simulink model "pmsm_control"  (R2018b)
settings: Solver=FixedStepDiscrete  StartTime=0.0  StopTime=0.5  FixedStep=dt_plant_sim  RelTol=1e-6  EnableMultiTasking=on
InitFcn:
  | pmsm_control_init
values from neighbouring files (symbols this model uses):
  D_safe = Simulink.Parameter(single(D0))    [pmsm_control_init.m]
  dt = 50e-9    (= 5e-08)    [pmsm_init.m]
  I_limit = Simulink.Parameter(single(Imax))    [pmsm_control_init.m]
  Id_Ki = Simulink.Parameter(single((Id_Kp.Value / TI) * Ts_current))    [pmsm_control_init.m]
  Id_Kp = Simulink.Parameter(single(wc * Ld))    [pmsm_control_init.m]
  ImaxFX = 600    [pmsm_init.m]
  Iq_Ki = Simulink.Parameter(single((Iq_Kp.Value / TI) * Ts_current))    [pmsm_control_init.m]
  Iq_Kp = Simulink.Parameter(single(wc * Lq))    [pmsm_control_init.m]
  J = Tst*Tau/W    (= 0.15)    [pmsm_init.m]
  L = Ld    [pmsm_control_init.m]    (also in pmsm_init.m = [Ld Lq])
  Ld = 0.37e-3    (= 0.00037)    [pmsm_init.m]
  Lq = 1.2e-3    (= 0.0012)    [pmsm_init.m]
  modulation_limit = Simulink.Parameter(single(0.577350269189626))    [pmsm_control_init.m]
  open_loop_iq_ref = Simulink.Parameter(single(5))    [pmsm_control_init.m]
  open_loop_mode = Simulink.Parameter(boolean(0))    [pmsm_control_init.m]
  pp = 3    [pmsm_init.m]
  Psi_PM = 66e-3    (= 0.066)    [pmsm_init.m]
  PsimaxFX = 2*abs(Psi_PM + Ld*Imax + j*Lq*Imax)    [pmsm_init.m]
  PWM_it_period = Simulink.Parameter(2)    [pmsm_control_init.m]
  R = 18e-3    (= 0.018)    [pmsm_init.m]
  Speed_Iq_limit = Simulink.Parameter(single(40))    [pmsm_control_init.m]
  Speed_Ki = Simulink.Parameter(single(Speed_Kp.Value / 0.03))    [pmsm_control_init.m]
  Speed_Kp = Simulink.Parameter(single(0.4))    [pmsm_control_init.m]
  TaumaxFX = (3/2)*pp*real(j*(Psi_PM + Ld*Imax + j*Lq*Imax)*Imax*(-1+j))    [pmsm_init.m]
  Ts = 1 / fsw    (= 0.0001)    [pmsm_control_init.m]
  Ts_current = Ts    (= 0.0001)    [pmsm_control_init.m]
  Ub = Udc / 2    [pmsm_control_init.m]
  Udc = 300    [pmsm_init.m]
  Udc_min = Simulink.Parameter(single(20))    [pmsm_control_init.m]
  UmaxFX = 600    [pmsm_init.m]
  WmaxFX = 1500*pp    (= 4500)    [pmsm_init.m]
undefined symbols (not defined in the file or in its folder): DiscIntNeverNeededParam, j
libraries: simulink x7
settings Model: ModifiedByFormat=The MathWorks Inc.  Creator=The MathWorks, Inc.  LastModifiedBy=The MathWorks Inc.
settings DataIOCC: LimitDataPoints=on  SaveFormat=Array  SaveOutput=off  SaveTime=off
settings OptimizationCC: ExpressionDepthLimit=2147483647  LifeSpan=1
settings DebuggingCC: MergeDetectMultiDrivingBlocksExec=none  SolverPrmCheckMsg=warning  FcnCallInpInsideContextMsg=warning  StateNameClashWarn=warning  SFUnexpectedBacktrackingDiag=warning  SFNoUnconditionalDefaultTransitionDiag=warning  SFExecutionAtInitializationDiag=none
settings HardwareCC: ProdBitPerPointer=32  ProdBitPerSizeT=32  ProdBitPerPtrDiffT=32  ProdLargestAtomicFloat=None  ProdIntDivRoundTo=Undefined  ProdEndianess=Unspecified  ProdWordSize=32  ProdHWDeviceType=32-bit Generic
settings ModelReferenceCC: PropagateSignalLabelsOutOfModel=off
settings SFSimCC: SimUseLocalCustomCode=off
settings RTWCC: RTWUseLocalCustomCode=off
settings CodeAppCC: StateflowObjectComments=on
settings GRTTargetCC: TargetLangStandard=C89/C90 (ANSI)  CombineOutputUpdateFcns=off  GRTInterface=on
settings ConfigComp: CovMetricSettings=dw  CovSaveCumulativeToWorkspaceVar=on  CovSaveSingleToWorkspaceVar=on  CovExternalEMLEnable=off  CovSFcnEnable=off

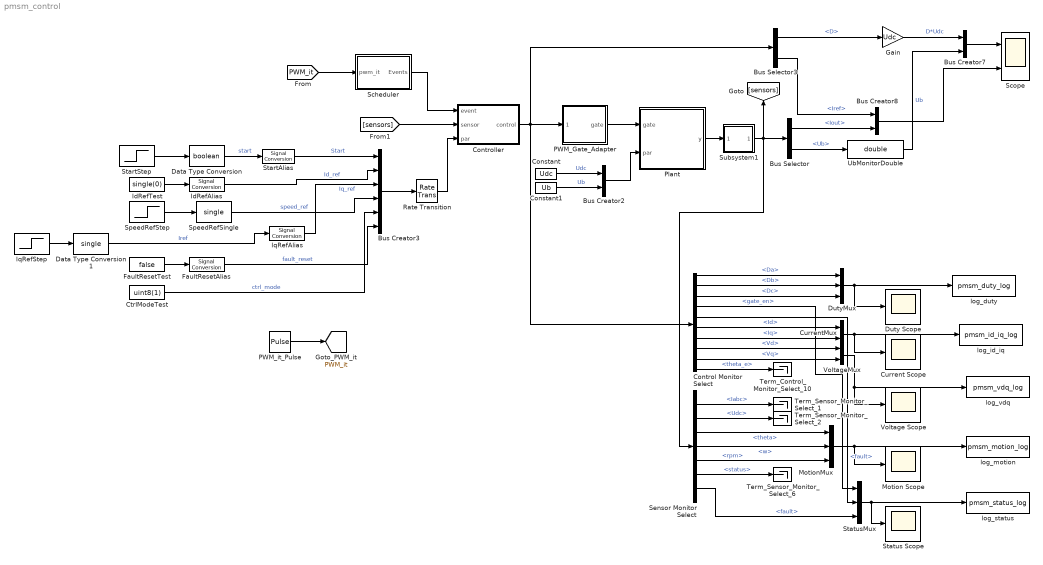
== system pmsm_control ==
  Bus Creator2 : BusCreator  Inputs=2
  Bus Creator3 : BusCreator  Inputs=6
  Bus Creator7 : BusCreator  Inputs=2
  Bus Creator8 : BusCreator  Inputs=2
  Bus Selector : BusSelector  OutputSignals=Iout,Ub
  Bus Selector3 : BusSelector  OutputSignals=D,Iref
  Constant : Constant  Value=Udc  SampleTime=-1
  Constant1 : Constant  Value=Ub  SampleTime=-1
  Control Monitor Select : BusSelector  OutputSignals=Da,Db,Dc,gate_en,fault,Id,Iq,Vd,Vq,theta_e
  Controller : Subsystem
  CtrlModeTest : Constant  Value=uint8(1)  OutDataTypeStr=uint8
  Current Scope : Scope
  CurrentMux : Mux  Inputs=2
  Data Type Conversion : DataTypeConversion  OutDataTypeStr=boolean
  Data Type Conversion1 : DataTypeConversion  OutDataTypeStr=single
  Duty Scope : Scope
  DutyMux : Mux  Inputs=3
  FaultResetAlias : SignalConversion  OverrideOpt=off
  FaultResetTest : Constant  Value=false  OutDataTypeStr=boolean
  Gain : Gain  Gain=Udc  ParamDataTypeStr=double  OutDataTypeStr=double
  IdRefAlias : SignalConversion  OverrideOpt=off
  IdRefTest : Constant  Value=single(0)  OutDataTypeStr=single
  IqRefAlias : SignalConversion  OverrideOpt=off
  IqRefStep : Step  Time=0  After=20  SampleTime=0
  Motion Scope : Scope
  MotionMux : Mux  Inputs=3
  PWM_Gate_Adapter : Subsystem
  PWM_it_Pulse : DiscretePulseGenerator  Period=PWM_it_period  SampleTime=Ts_current/2
  Plant : Subsystem
  Rate Transition : RateTransition  Integrity=off  Deterministic=off
  Scheduler : Subsystem
  Scope : Scope  NumInputPorts=2
  Sensor Monitor Select : BusSelector  OutputSignals=Iabc,Udc,theta,w,rpm,status,fault
  SpeedRefSingle : DataTypeConversion  OutDataTypeStr=single
  SpeedRefStep : Step  Time=0  Before=100  After=100  SampleTime=0
  StartAlias : SignalConversion  OverrideOpt=off
  StartStep : Step  Time=0  SampleTime=0
  Status Scope : Scope
  StatusMux : Mux  Inputs=3
  Subsystem1 : Subsystem
  Term_Control_Monitor_Select_10 : Terminator
  Term_Sensor_Monitor_Select_1 : Terminator
  Term_Sensor_Monitor_Select_2 : Terminator
  Term_Sensor_Monitor_Select_6 : Terminator
  UbMonitorDouble : DataTypeConversion  OutDataTypeStr=double
  Voltage Scope : Scope
  VoltageMux : Mux  Inputs=2
  log_duty : ToWorkspace  VariableName=pmsm_duty_log  SaveFormat=Structure With Time  SampleTime=-1
  log_id_iq : ToWorkspace  VariableName=pmsm_id_iq_log  SaveFormat=Structure With Time  SampleTime=-1
  log_motion : ToWorkspace  VariableName=pmsm_motion_log  SaveFormat=Structure With Time  SampleTime=-1
  log_status : ToWorkspace  VariableName=pmsm_status_log  SaveFormat=Structure With Time  SampleTime=-1
  log_vdq : ToWorkspace  VariableName=pmsm_vdq_log  SaveFormat=Structure With Time  SampleTime=-1
  tag scope: PWM_it=global
  wires:
  Constant/1 -> Bus Creator2/1  "Udc"
  Constant1/1 -> Bus Creator2/2  "Ub"
  Bus Selector3/1 -> Gain/1  "<D>"
  Gain/1 -> Bus Creator7/1  "D*Udc"
  Bus Selector3/2 -> Bus Creator8/1  "<Iref>"
  Bus Selector/1 -> Bus Creator8/2  "<Iout>"
  Bus Creator7/1 -> Scope/1
  Bus Creator8/1 -> Scope/2
  Scheduler/1(Events) -> Controller/1(event)
  Data Type Conversion/1 -> StartAlias/1  "start"
  Data Type Conversion1/1 -> IqRefAlias/1  "Iref"
  Bus Creator3/1 -> Rate Transition/1
  [sensors] -> Controller/2(sensor)
  Subsystem1/1(Out1) -> Sensor Monitor Select/1, Bus Selector/1, [sensors]
  Rate Transition/1 -> Controller/3(par)
  [PWM_it] -> Scheduler/1(pwm_it)
  IdRefTest/1 -> IdRefAlias/1
  FaultResetTest/1 -> FaultResetAlias/1
  DutyMux/1 -> log_duty/1, Duty Scope/1
  CurrentMux/1 -> Current Scope/1, log_id_iq/1
  VoltageMux/1 -> Voltage Scope/1, log_vdq/1
  MotionMux/1 -> Motion Scope/1, log_motion/1
  StatusMux/1 -> Status Scope/1, log_status/1
  StartStep/1 -> Data Type Conversion/1
  IqRefStep/1 -> Data Type Conversion1/1
  Control Monitor Select/1 -> DutyMux/1  "<Da>"
  Control Monitor Select/2 -> DutyMux/2  "<Db>"
  Control Monitor Select/3 -> DutyMux/3  "<Dc>"
  Control Monitor Select/6 -> CurrentMux/1  "<Id>"
  Control Monitor Select/7 -> CurrentMux/2  "<Iq>"
  Control Monitor Select/8 -> VoltageMux/1  "<Vd>"
  Control Monitor Select/9 -> VoltageMux/2  "<Vq>"
  Sensor Monitor Select/3 -> MotionMux/1  "<theta>"
  Sensor Monitor Select/4 -> MotionMux/2  "<w>"
  Sensor Monitor Select/5 -> MotionMux/3  "<rpm>"
  Control Monitor Select/4 -> StatusMux/1  "<gate_en>"
  Control Monitor Select/5 -> StatusMux/2  "<fault>"
  Sensor Monitor Select/7 -> StatusMux/3  "<fault>"
  Bus Selector/2 -> UbMonitorDouble/1  "<Ub>"
  UbMonitorDouble/1 -> Bus Creator7/2  "Ub"
  Controller/1(control) -> PWM_Gate_Adapter/1(control), Bus Selector3/1, Control Monitor Select/1
  Control Monitor Select/10 -> Term_Control_Monitor_Select_10/1  "<theta_e>"
  Sensor Monitor Select/1 -> Term_Sensor_Monitor_Select_1/1  "<Iabc>"
  Sensor Monitor Select/2 -> Term_Sensor_Monitor_Select_2/1  "<Udc>"
  Sensor Monitor Select/6 -> Term_Sensor_Monitor_Select_6/1  "<status>"
  PWM_Gate_Adapter/1(gate) -> Plant/1(gate)
  Bus Creator2/1 -> Plant/2(par)
  Plant/1(y) -> Subsystem1/1(In1)
  StartAlias/1 -> Bus Creator3/1  "Start"
  IdRefAlias/1 -> Bus Creator3/2  "Id_ref"
  IqRefAlias/1 -> Bus Creator3/3  "Iq_ref"
  FaultResetAlias/1 -> Bus Creator3/6  "fault_reset"
  PWM_it_Pulse/1 -> [PWM_it]
  SpeedRefStep/1 -> SpeedRefSingle/1
  SpeedRefSingle/1 -> Bus Creator3/4  "speed_ref"
  CtrlModeTest/1 -> Bus Creator3/5  "ctrl_mode"

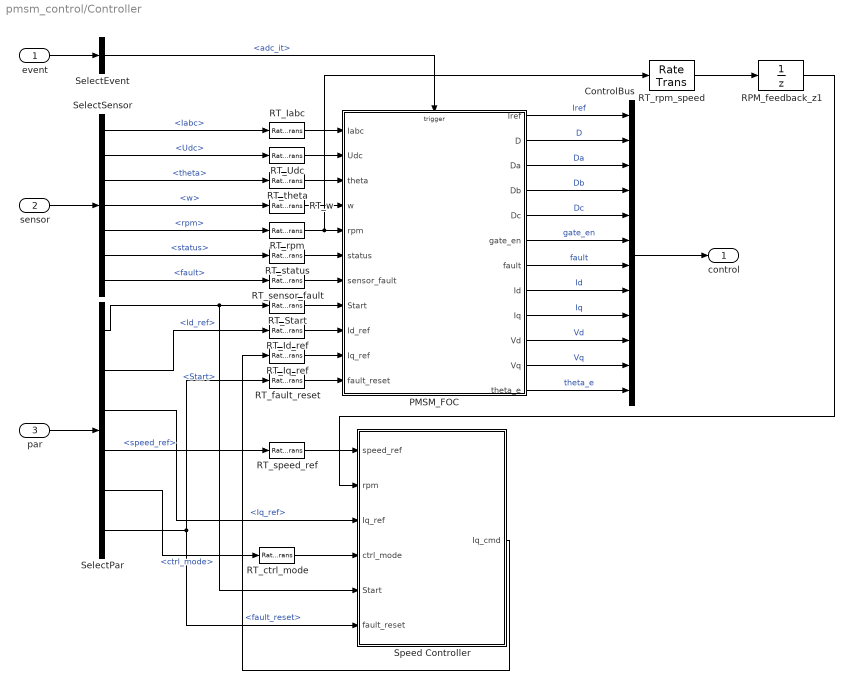
== system pmsm_control/Controller ==
  event : Inport
  sensor : Inport  Port=2
  par : Inport  Port=3
  ControlBus : BusCreator  Inputs=12
  PMSM_FOC : Subsystem  TreatAsAtomicUnit=on
  RPM_feedback_z1 : UnitDelay  InitialCondition=single(0)  SampleTime=-1
  RT_Iabc : RateTransition  Integrity=off  Deterministic=off  OutPortSampleTimeOpt=Inherit
  RT_Id_ref : RateTransition  Integrity=off  Deterministic=off  OutPortSampleTimeOpt=Inherit
  RT_Iq_ref : RateTransition  Integrity=off  Deterministic=off  OutPortSampleTimeOpt=Inherit
  RT_Start : RateTransition  Integrity=off  Deterministic=off  OutPortSampleTimeOpt=Inherit
  RT_Udc : RateTransition  Integrity=off  Deterministic=off  OutPortSampleTimeOpt=Inherit
  RT_ctrl_mode : RateTransition  Integrity=off  Deterministic=off  OutPortSampleTimeOpt=Inherit
  RT_fault_reset : RateTransition  Integrity=off  Deterministic=off  OutPortSampleTimeOpt=Inherit
  RT_rpm : RateTransition  Integrity=off  Deterministic=off  OutPortSampleTimeOpt=Inherit
  RT_rpm_speed : RateTransition  Deterministic=off  OutPortSampleTimeOpt=Inherit
  RT_sensor_fault : RateTransition  Integrity=off  Deterministic=off  OutPortSampleTimeOpt=Inherit
  RT_speed_ref : RateTransition  Integrity=off  Deterministic=off  OutPortSampleTimeOpt=Inherit
  RT_status : RateTransition  Integrity=off  Deterministic=off  OutPortSampleTimeOpt=Inherit
  RT_theta : RateTransition  Integrity=off  Deterministic=off  OutPortSampleTimeOpt=Inherit
  RT_w : RateTransition  Integrity=off  Deterministic=off  OutPortSampleTimeOpt=Inherit
  SelectEvent : BusSelector  OutputSignals=interrupts.adc_it
  SelectPar : BusSelector  OutputSignals=Start,Id_ref,Iq_ref,speed_ref,ctrl_mode,fault_reset
  SelectSensor : BusSelector  OutputSignals=Iabc,Udc,theta,w,rpm,status,fault
  Speed Controller : Subsystem
  control : Outport
  wires:
  RPM_feedback_z1/1 -> Speed Controller/2(rpm)
  RT_rpm_speed/1 -> RPM_feedback_z1/1
  PMSM_FOC/12(theta_e) -> ControlBus/12  "theta_e"
  PMSM_FOC/11(Vq) -> ControlBus/11  "Vq"
  PMSM_FOC/10(Vd) -> ControlBus/10  "Vd"
  PMSM_FOC/9(Iq) -> ControlBus/9  "Iq"
  PMSM_FOC/8(Id) -> ControlBus/8  "Id"
  PMSM_FOC/7(fault) -> ControlBus/7  "fault"
  PMSM_FOC/6(gate_en) -> ControlBus/6  "gate_en"
  PMSM_FOC/5(Dc) -> ControlBus/5  "Dc"
  PMSM_FOC/4(Db) -> ControlBus/4  "Db"
  PMSM_FOC/3(Da) -> ControlBus/3  "Da"
  PMSM_FOC/2(D) -> ControlBus/2  "D"
  PMSM_FOC/1(Iref) -> ControlBus/1  "Iref"
  RT_fault_reset/1 -> PMSM_FOC/11(fault_reset)
  RT_Iq_ref/1 -> PMSM_FOC/10(Iq_ref)
  RT_Id_ref/1 -> PMSM_FOC/9(Id_ref)
  RT_Start/1 -> PMSM_FOC/8(Start)
  RT_sensor_fault/1 -> PMSM_FOC/7(sensor_fault)
  RT_status/1 -> PMSM_FOC/6(status)
  RT_rpm/1 -> RT_rpm_speed/1, PMSM_FOC/5(rpm)
  RT_w/1 -> PMSM_FOC/4(w)
  RT_theta/1 -> PMSM_FOC/3(theta)
  RT_Udc/1 -> PMSM_FOC/2(Udc)
  RT_Iabc/1 -> PMSM_FOC/1(Iabc)
  ControlBus/1 -> control/1
  SelectSensor/7 -> RT_sensor_fault/1  "<fault>"
  SelectSensor/6 -> RT_status/1  "<status>"
  SelectSensor/5 -> RT_rpm/1  "<rpm>"
  SelectSensor/4 -> RT_w/1  "<w>"
  SelectSensor/3 -> RT_theta/1  "<theta>"
  SelectSensor/2 -> RT_Udc/1  "<Udc>"
  SelectSensor/1 -> RT_Iabc/1  "<Iabc>"
  SelectEvent/1 -> PMSM_FOC/Trigger  "<adc_it>"
  par/1 -> SelectPar/1
  sensor/1 -> SelectSensor/1
  event/1 -> SelectEvent/1
  SelectPar/1 -> Speed Controller/5(Start), RT_Start/1  "<Start>"
  SelectPar/2 -> RT_Id_ref/1  "<Id_ref>"
  SelectPar/3 -> Speed Controller/3(Iq_ref)  "<Iq_ref>"
  SelectPar/4 -> RT_speed_ref/1  "<speed_ref>"
  SelectPar/5 -> RT_ctrl_mode/1  "<ctrl_mode>"
  SelectPar/6 -> Speed Controller/6(fault_reset), RT_fault_reset/1  "<fault_reset>"
  RT_speed_ref/1 -> Speed Controller/1(speed_ref)
  RT_ctrl_mode/1 -> Speed Controller/4(ctrl_mode)
  Speed Controller/1(Iq_cmd) -> RT_Iq_ref/1

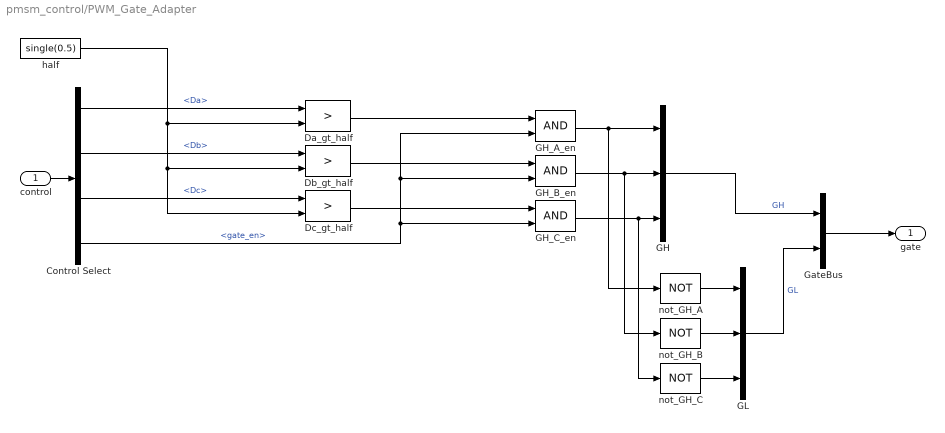
== system pmsm_control/PWM_Gate_Adapter ==
  control : Inport
  Control Select : BusSelector  OutputSignals=Da,Db,Dc,gate_en
  Da_gt_half : RelationalOperator  Operator=>  OutDataTypeStr=boolean  RndMeth=Simplest
  Db_gt_half : RelationalOperator  Operator=>  OutDataTypeStr=boolean  RndMeth=Simplest
  Dc_gt_half : RelationalOperator  Operator=>  OutDataTypeStr=boolean  RndMeth=Simplest
  GH : Mux  Inputs=3
  GH_A_en : Logic  AllPortsSameDT=off  OutDataTypeStr=boolean
  GH_B_en : Logic  AllPortsSameDT=off  OutDataTypeStr=boolean
  GH_C_en : Logic  AllPortsSameDT=off  OutDataTypeStr=boolean
  GL : Mux  Inputs=3
  GateBus : BusCreator  Inputs=2
  half : Constant  Value=single(0.5)  OutDataTypeStr=single
  not_GH_A : Logic  Operator=NOT  AllPortsSameDT=off  OutDataTypeStr=boolean
  not_GH_B : Logic  Operator=NOT  AllPortsSameDT=off  OutDataTypeStr=boolean
  not_GH_C : Logic  Operator=NOT  AllPortsSameDT=off  OutDataTypeStr=boolean
  gate : Outport
  wires:
  Control Select/1 -> Da_gt_half/1  "<Da>"
  half/1 -> Da_gt_half/2, Dc_gt_half/2, Db_gt_half/2
  Da_gt_half/1 -> GH_A_en/1
  Control Select/4 -> GH_A_en/2, GH_B_en/2, GH_C_en/2  "<gate_en>"
  GH_A_en/1 -> GH/1, not_GH_A/1
  Control Select/2 -> Db_gt_half/1  "<Db>"
  Db_gt_half/1 -> GH_B_en/1
  GH_B_en/1 -> GH/2, not_GH_B/1
  Control Select/3 -> Dc_gt_half/1  "<Dc>"
  Dc_gt_half/1 -> GH_C_en/1
  GH_C_en/1 -> not_GH_C/1, GH/3
  control/1 -> Control Select/1
  not_GH_A/1 -> GL/1
  not_GH_B/1 -> GL/2
  not_GH_C/1 -> GL/3
  GH/1 -> GateBus/1  "GH"
  GL/1 -> GateBus/2  "GL"
  GateBus/1 -> gate/1

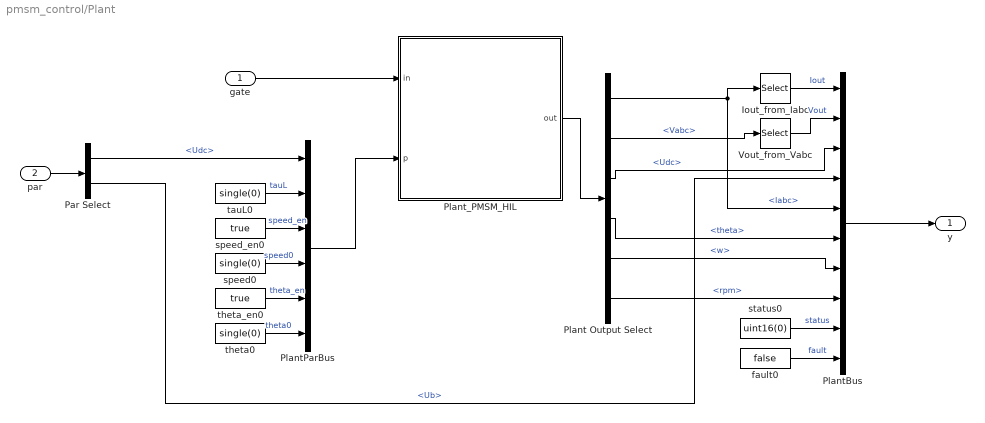
== system pmsm_control/Plant ==
  gate : Inport
  par : Inport  Port=2
  Iout_from_Iabc : Selector  InputPortWidth=3  IndexOptions=Index vector (dialog)  Indices=1  OutputSizes=1
  Par Select : BusSelector  OutputSignals=Udc,Ub
  Plant Output Select : BusSelector  OutputSignals=Iabc,Vabc,Udc,theta,w,rpm
  PlantBus : BusCreator  Inputs=10
  PlantParBus : BusCreator  Inputs=6
  Plant_PMSM_HIL : Subsystem
  Vout_from_Vabc : Selector  InputPortWidth=3  IndexOptions=Index vector (dialog)  Indices=1  OutputSizes=1
  fault0 : Constant  Value=false  OutDataTypeStr=boolean
  speed0 : Constant  Value=single(0)  OutDataTypeStr=single
  speed_en0 : Constant  Value=true  OutDataTypeStr=boolean
  status0 : Constant  Value=uint16(0)  OutDataTypeStr=uint16
  tauL0 : Constant  Value=single(0)  OutDataTypeStr=single
  theta0 : Constant  Value=single(0)  OutDataTypeStr=single
  theta_en0 : Constant  Value=true  OutDataTypeStr=boolean
  y : Outport
  wires:
  Par Select/1 -> PlantParBus/1  "<Udc>"
  tauL0/1 -> PlantParBus/2  "tauL"
  speed_en0/1 -> PlantParBus/3  "speed_en"
  speed0/1 -> PlantParBus/4  "speed0"
  theta_en0/1 -> PlantParBus/5  "theta_en"
  theta0/1 -> PlantParBus/6  "theta0"
  Plant Output Select/1 -> Iout_from_Iabc/1, PlantBus/5  "<Iabc>"
  Plant Output Select/2 -> Vout_from_Vabc/1  "<Vabc>"
  Iout_from_Iabc/1 -> PlantBus/1  "Iout"
  Vout_from_Vabc/1 -> PlantBus/2  "Vout"
  Plant Output Select/3 -> PlantBus/3  "<Udc>"
  Par Select/2 -> PlantBus/4  "<Ub>"
  Plant Output Select/4 -> PlantBus/6  "<theta>"
  Plant Output Select/5 -> PlantBus/7  "<w>"
  Plant Output Select/6 -> PlantBus/8  "<rpm>"
  status0/1 -> PlantBus/9  "status"
  fault0/1 -> PlantBus/10  "fault"
  gate/1 -> Plant_PMSM_HIL/1(in)
  par/1 -> Par Select/1
  PlantParBus/1 -> Plant_PMSM_HIL/2(p)
  Plant_PMSM_HIL/1(out) -> Plant Output Select/1
  PlantBus/1 -> y/1

== system pmsm_control/Scheduler ==
  pwm_it : Inport
  AsynchronousScheduler : Stateflow chart  TreatAsAtomicUnit=on
      settings: RTWMemSecFuncInitTerm=Default  RTWMemSecFuncExecute=Default
  Bus Creator : BusCreator  Inputs=1
  Bus Creator4 : BusCreator  Inputs=2
  Bus Creator5 : BusCreator  Inputs=3
  Function-Call Generator : simulink/Ports & Subsystems/Function-Call Generator  sample_time=1e-3  numberOfIterations=1
  Function-Call Generator1 : simulink/Ports & Subsystems/Function-Call Generator  sample_time=100e-3  numberOfIterations=1
  Function-Call Generator2 : simulink/Ports & Subsystems/Function-Call Generator  sample_time=1  numberOfIterations=1
  Events : Outport
  wires:
  Bus Creator5/1 -> Bus Creator4/2  "timers"
  Function-Call Generator2/1 -> Bus Creator5/3  "T_1s"
  Bus Creator/1 -> Bus Creator4/1  "interrupts"
  pwm_it/1 -> AsynchronousScheduler/Trigger  "pwm_it"
  AsynchronousScheduler/1(adc_it()) -> Bus Creator/1
  Bus Creator4/1 -> Events/1
  Function-Call Generator1/1 -> Bus Creator5/2  "T_100ms"
  Function-Call Generator/1 -> Bus Creator5/1  "T_1ms"

== system pmsm_control/Subsystem1 ==
  In1 : Inport
  Iabc_conv : DataTypeConversion  OutDataTypeStr=single
  Iout_conv : DataTypeConversion  OutDataTypeStr=single
  SelectPlant : BusSelector  OutputSignals=Iout,Vout,Udc,Ub,Iabc,theta,w,rpm,status,fault
  SensorBus : BusCreator  Inputs=10
  Ub_conv : DataTypeConversion  OutDataTypeStr=single
  Udc_conv : DataTypeConversion  OutDataTypeStr=single
  Vout_conv : DataTypeConversion  OutDataTypeStr=single
  fault_conv : DataTypeConversion  OutDataTypeStr=boolean
  rpm_conv : DataTypeConversion  OutDataTypeStr=single
  status_conv : DataTypeConversion  OutDataTypeStr=uint16
  theta_conv : DataTypeConversion  OutDataTypeStr=single
  w_conv : DataTypeConversion  OutDataTypeStr=single
  Out1 : Outport
  wires:
  In1/1 -> SelectPlant/1
  SelectPlant/1 -> Iout_conv/1  "<Iout>"
  Iout_conv/1 -> SensorBus/1  "Iout"
  SelectPlant/2 -> Vout_conv/1  "<Vout>"
  Vout_conv/1 -> SensorBus/2  "Vout"
  SelectPlant/3 -> Udc_conv/1  "<Udc>"
  Udc_conv/1 -> SensorBus/3  "Udc"
  SelectPlant/4 -> Ub_conv/1  "<Ub>"
  Ub_conv/1 -> SensorBus/4  "Ub"
  SelectPlant/5 -> Iabc_conv/1  "<Iabc>"
  Iabc_conv/1 -> SensorBus/5  "Iabc"
  SelectPlant/6 -> theta_conv/1  "<theta>"
  theta_conv/1 -> SensorBus/6  "theta"
  SelectPlant/7 -> w_conv/1  "<w>"
  w_conv/1 -> SensorBus/7  "w"
  SelectPlant/8 -> rpm_conv/1  "<rpm>"
  rpm_conv/1 -> SensorBus/8  "rpm"
  SelectPlant/9 -> status_conv/1  "<status>"
  status_conv/1 -> SensorBus/9  "status"
  SelectPlant/10 -> fault_conv/1  "<fault>"
  fault_conv/1 -> SensorBus/10  "fault"
  SensorBus/1 -> Out1/1

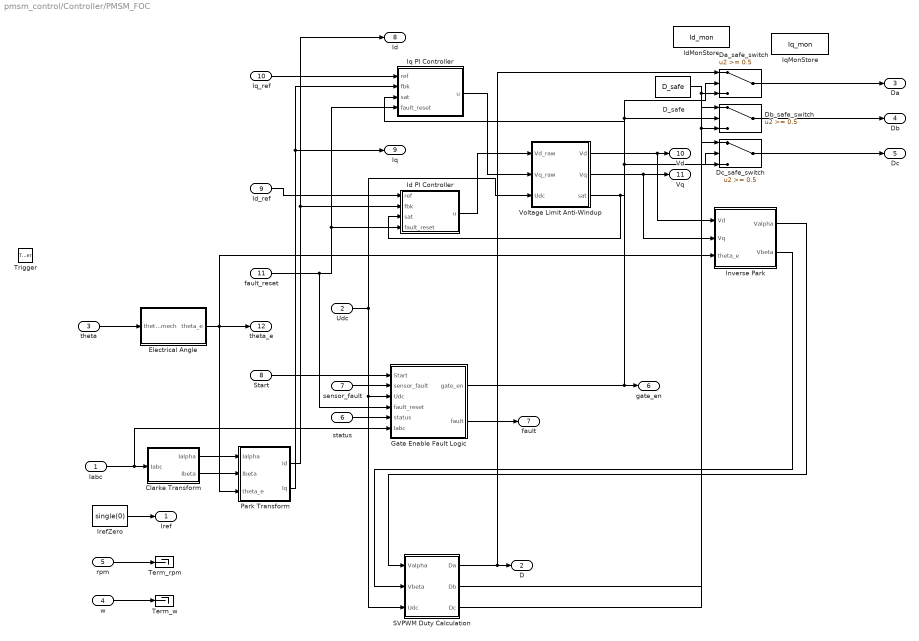
== system pmsm_control/Controller/PMSM_FOC ==
  Iabc : Inport
  Udc : Inport  Port=2
  theta : Inport  Port=3
  w : Inport  Port=4
  rpm : Inport  Port=5
  status : Inport  Port=6
  sensor_fault : Inport  Port=7
  Start : Inport  Port=8
  Id_ref : Inport  Port=9
  Iq_ref : Inport  Port=10
  fault_reset : Inport  Port=11
  Trigger : TriggerPort  TriggerType=function-call  VariantControl=Variant
  Clarke Transform : Subsystem
  D_safe : Constant  Value=D_safe  SampleTime=-1
  Da_safe_switch : Switch  Threshold=0.5
  Db_safe_switch : Switch  Threshold=0.5
  Dc_safe_switch : Switch  Threshold=0.5
  Electrical Angle : Subsystem
  Gate Enable Fault Logic : Subsystem
  Id PI Controller : Subsystem
  IdMonStore : DataStoreMemory  DataStoreName=Id_mon  ReadBeforeWriteMsg=warning  WriteAfterWriteMsg=warning  WriteAfterReadMsg=warning  InitialValue=single(0)  ShowAdditionalParam=off  OutDataTypeStr=single
      settings: RTWStateStorageClass=ExportedGlobal
  Inverse Park : Subsystem
  Iq PI Controller : Subsystem
  IqMonStore : DataStoreMemory  DataStoreName=Iq_mon  ReadBeforeWriteMsg=warning  WriteAfterWriteMsg=warning  WriteAfterReadMsg=warning  InitialValue=single(0)  ShowAdditionalParam=off  OutDataTypeStr=single
      settings: RTWStateStorageClass=ExportedGlobal
  IrefZero : Constant  Value=single(0)  OutDataTypeStr=single  SampleTime=-1
  Park Transform : Subsystem
  SVPWM Duty Calculation : Subsystem
  Term_rpm : Terminator
  Term_w : Terminator
  Voltage Limit Anti-Windup : Subsystem
  Iref : Outport
  D : Outport  Port=2
  Da : Outport  Port=3
  Db : Outport  Port=4
  Dc : Outport  Port=5
  gate_en : Outport  Port=6
  fault : Outport  Port=7
  Id : Outport  Port=8
  Iq : Outport  Port=9
  Vd : Outport  Port=10
  Vq : Outport  Port=11
  theta_e : Outport  Port=12
  wires:
  Dc_safe_switch/1 -> Dc/1
  Db_safe_switch/1 -> Db/1
  Da_safe_switch/1 -> Da/1
  SVPWM Duty Calculation/3(Dc) -> Dc_safe_switch/1
  SVPWM Duty Calculation/2(Db) -> Db_safe_switch/1
  status/1 -> Gate Enable Fault Logic/5(status)
  SVPWM Duty Calculation/1(Da) -> Da_safe_switch/1, D/1
  Electrical Angle/1(theta_e) -> Inverse Park/3(theta_e), theta_e/1, Park Transform/3(theta_e)
  D_safe/1 -> Dc_safe_switch/3, Db_safe_switch/3, Da_safe_switch/3
  Voltage Limit Anti-Windup/1(Vd) -> Vd/1, Inverse Park/1(Vd)
  Voltage Limit Anti-Windup/3(sat) -> Iq PI Controller/3(sat), Id PI Controller/3(sat)
  Iabc/1 -> Gate Enable Fault Logic/6(Iabc), Clarke Transform/1(Iabc)
  Park Transform/1(Id) -> Id/1, Id PI Controller/2(fbk)
  Park Transform/2(Iq) -> Iq/1, Iq PI Controller/2(fbk)
  Udc/1 -> SVPWM Duty Calculation/3(Udc), Gate Enable Fault Logic/3(Udc), Voltage Limit Anti-Windup/3(Udc)
  Voltage Limit Anti-Windup/2(Vq) -> Vq/1, Inverse Park/2(Vq)
  fault_reset/1 -> Iq PI Controller/4(fault_reset), Id PI Controller/4(fault_reset), Gate Enable Fault Logic/4(fault_reset)
  Gate Enable Fault Logic/1(gate_en) -> Db_safe_switch/2, Da_safe_switch/2, Dc_safe_switch/2, gate_en/1
  theta/1 -> Electrical Angle/1(theta_mech)
  Clarke Transform/1(Ialpha) -> Park Transform/1(Ialpha)
  Clarke Transform/2(Ibeta) -> Park Transform/2(Ibeta)
  Id PI Controller/1(u) -> Voltage Limit Anti-Windup/1(Vd_raw)
  Iq PI Controller/1(u) -> Voltage Limit Anti-Windup/2(Vq_raw)
  Id_ref/1 -> Id PI Controller/1(ref)
  Iq_ref/1 -> Iq PI Controller/1(ref)
  Inverse Park/1(Valpha) -> SVPWM Duty Calculation/1(Valpha)
  Inverse Park/2(Vbeta) -> SVPWM Duty Calculation/2(Vbeta)
  Start/1 -> Gate Enable Fault Logic/1(Start)
  sensor_fault/1 -> Gate Enable Fault Logic/2(sensor_fault)
  IrefZero/1 -> Iref/1
  Gate Enable Fault Logic/2(fault) -> fault/1
  w/1 -> Term_w/1
  rpm/1 -> Term_rpm/1

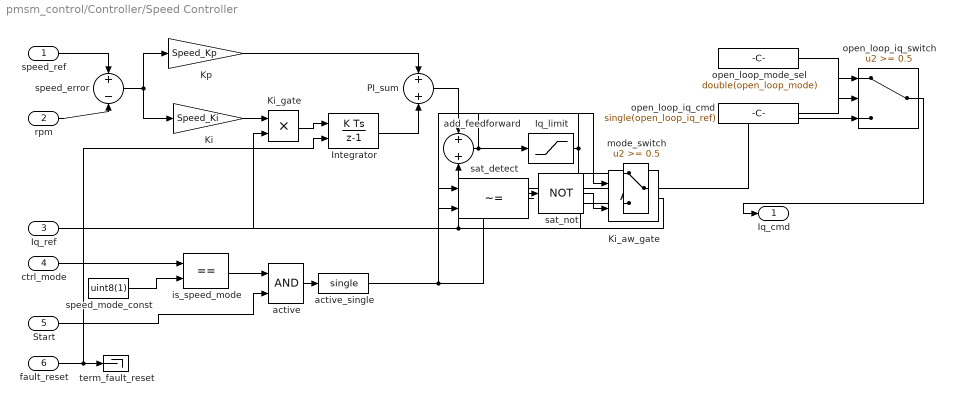
== system pmsm_control/Controller/Speed Controller ==
  speed_ref : Inport
  rpm : Inport  Port=2
  Iq_ref : Inport  Port=3
  ctrl_mode : Inport  Port=4
  Start : Inport  Port=5
  fault_reset : Inport  Port=6
  Integrator : DiscreteIntegrator  ExternalReset=rising  InitialCondition=single(0)  SampleTime=-1  ICPrevOutput=DiscIntNeverNeededParam  ICPrevScaledInput=DiscIntNeverNeededParam
  Iq_limit : Saturate  UpperLimit=Speed_Iq_limit  LowerLimit=-Speed_Iq_limit
  Ki : Gain  Gain=Speed_Ki
  Ki_aw_gate : Logic  AllPortsSameDT=off  OutDataTypeStr=boolean
  Ki_gate : Product  Inputs=**
  Kp : Gain  Gain=Speed_Kp
  PI_sum : Sum
  active : Logic  AllPortsSameDT=off  OutDataTypeStr=boolean
  active_single : DataTypeConversion  OutDataTypeStr=single
  add_feedforward : Sum
  is_speed_mode : RelationalOperator  Operator===  OutDataTypeStr=boolean  RndMeth=Simplest
  mode_switch : Switch  Threshold=0.5
  open_loop_iq_cmd : Constant  Value=single(open_loop_iq_ref)
  open_loop_iq_switch : Switch  Threshold=0.5
  open_loop_mode_sel : Constant  Value=double(open_loop_mode)
  sat_detect : RelationalOperator  Operator=~=  OutDataTypeStr=boolean  RndMeth=Simplest
  sat_not : Logic  Operator=NOT  AllPortsSameDT=off  OutDataTypeStr=boolean
  speed_error : Sum  Inputs=+-
  speed_mode_const : Constant  Value=uint8(1)  OutDataTypeStr=uint8
  term_fault_reset : Terminator
  Iq_cmd : Outport
  wires:
  open_loop_iq_switch/1 -> Iq_cmd/1
  open_loop_iq_cmd/1 -> open_loop_iq_switch/1
  open_loop_mode_sel/1 -> open_loop_iq_switch/2
  mode_switch/1 -> open_loop_iq_switch/3
  Ki_aw_gate/1 -> Ki_gate/2
  sat_not/1 -> Ki_aw_gate/2
  sat_detect/1 -> sat_not/1
  speed_ref/1 -> speed_error/1
  rpm/1 -> speed_error/2
  speed_error/1 -> Ki/1, Kp/1
  Ki/1 -> Ki_gate/1
  active_single/1 -> Ki_aw_gate/1, mode_switch/2
  Ki_gate/1 -> Integrator/1
  Kp/1 -> PI_sum/1
  Integrator/1 -> PI_sum/2
  PI_sum/1 -> add_feedforward/1
  Iq_ref/1 -> add_feedforward/2, mode_switch/3
  add_feedforward/1 -> sat_detect/1, Iq_limit/1
  ctrl_mode/1 -> is_speed_mode/1
  speed_mode_const/1 -> is_speed_mode/2
  is_speed_mode/1 -> active/1
  Start/1 -> active/2
  active/1 -> active_single/1
  Iq_limit/1 -> sat_detect/2, mode_switch/1
  fault_reset/1 -> Integrator/2, term_fault_reset/1

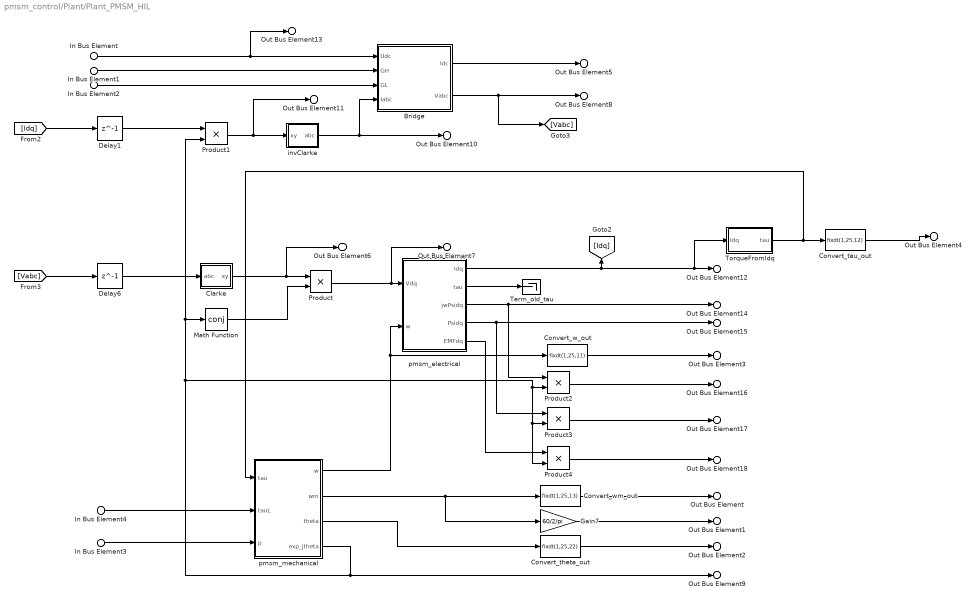
== system pmsm_control/Plant/Plant_PMSM_HIL ==
  In Bus Element1 : Inport  PortName=in  Element=GH
  In Bus Element2 : Inport  PortName=in  Element=GL
  In Bus Element3 : Inport  Port=2  PortName=p
  In Bus Element : Inport  Port=2  PortName=p  Element=Udc
  In Bus Element4 : Inport  Port=2  PortName=p  Element=tauL
  Bridge : Subsystem
  Clarke : Subsystem
  Convert_tau_out : DataTypeConversion  OutDataTypeStr=fixdt(1,25,12)
  Convert_theta_out : DataTypeConversion  OutDataTypeStr=fixdt(1,25,22)
  Convert_w_out : DataTypeConversion  OutDataTypeStr=fixdt(1,25,11)
  Convert_wm_out : DataTypeConversion  OutDataTypeStr=fixdt(1,25,13)
  Delay1 : Delay  DelayLength=1  InitialCondition=0
  Delay6 : Delay  DelayLength=1  InitialCondition=0
  Gain7 : Gain  Gain=60/2/pi  OutMax=[WmaxFX/pp*60/2/pi]  OutDataTypeStr=fixdt(1,vbits)
  Math Function : Math  Operator=conj  SaturateOnIntegerOverflow=on
  Product{,1..4} (5 alike) : Product  OutDataTypeStr=Inherit: Same as first input
  Term_old_tau : Terminator
  TorqueFromIdq : Subsystem
  invClarke : Subsystem
  pmsm_electrical : Subsystem
  pmsm_mechanical : Subsystem
  Out Bus Element : Outport  PortName=out  Element=wm
  Out Bus Element1 : Outport  PortName=out  Element=rpm
  Out Bus Element2 : Outport  PortName=out  Element=theta
  Out Bus Element3 : Outport  PortName=out  Element=w
  Out Bus Element4 : Outport  PortName=out  Element=tau
  Out Bus Element5 : Outport  PortName=out  Element=Idc
  Out Bus Element6 : Outport  PortName=out  Element=Vxy
  Out Bus Element7 : Outport  PortName=out  Element=Vdq
  Out Bus Element8 : Outport  PortName=out  Element=Vabc
  Out Bus Element9 : Outport  PortName=out  Element=exp_jtheta
  Out Bus Element10 : Outport  PortName=out  Element=Iabc
  Out Bus Element11 : Outport  PortName=out  Element=Ixy
  Out Bus Element12 : Outport  PortName=out  Element=Idq
  Out Bus Element13 : Outport  PortName=out  Element=Udc
  Out Bus Element14 : Outport  PortName=out  Element=jwPsidq
  Out Bus Element15 : Outport  PortName=out  Element=Psidq
  Out Bus Element16 : Outport  PortName=out  Element=jwPsixy
  Out Bus Element17 : Outport  PortName=out  Element=Psixy
  Out Bus Element18 : Outport  PortName=out  Element=EMFxy
  wires:
  invClarke/1(abc) -> Bridge/4(Iabc), Out Bus Element10/1
  Product1/1 -> Out Bus Element11/1, invClarke/1(xy)
  [Vabc] -> Delay6/1
  pmsm_mechanical/1(w) -> Convert_w_out/1, pmsm_electrical/2(w)
  Product/1 -> pmsm_electrical/1(Vdq), Out Bus Element7/1
  pmsm_electrical/1(Idq) -> [Idq], Out Bus Element12/1, TorqueFromIdq/1(Idq)
  [Idq] -> Delay1/1
  pmsm_mechanical/4(exp_jtheta) -> Out Bus Element9/1, Product4/2, Product3/2, Product2/2, Math Function/1, Product1/2
  Bridge/2(Vabc) -> [Vabc], Out Bus Element8/1
  Math Function/1 -> Product/2
  Clarke/1(xy) -> Product/1, Out Bus Element6/1
  Bridge/1(Idc) -> Out Bus Element5/1
  In Bus Element4/1 -> pmsm_mechanical/2(tauL)
  In Bus Element3/1 -> pmsm_mechanical/3(p)
  pmsm_mechanical/2(wm) -> Gain7/1, Convert_wm_out/1
  Gain7/1 -> Out Bus Element1/1
  In Bus Element2/1 -> Bridge/3(GL)
  In Bus Element1/1 -> Bridge/2(GH)
  In Bus Element/1 -> Out Bus Element13/1, Bridge/1(Udc)
  Delay1/1 -> Product1/1
  Delay6/1 -> Clarke/1(abc)
  pmsm_electrical/3(jwPsidq) -> Out Bus Element14/1, Product2/1
  pmsm_electrical/4(Psidq) -> Out Bus Element15/1, Product3/1
  Product2/1 -> Out Bus Element16/1
  Product3/1 -> Out Bus Element17/1
  pmsm_electrical/5(EMFdq) -> Product4/1
  Product4/1 -> Out Bus Element18/1
  TorqueFromIdq/1(tau) -> Convert_tau_out/1, pmsm_mechanical/1(tau)
  pmsm_electrical/2(tau) -> Term_old_tau/1
  Convert_wm_out/1 -> Out Bus Element/1
  pmsm_mechanical/3(theta) -> Convert_theta_out/1
  Convert_theta_out/1 -> Out Bus Element2/1
  Convert_w_out/1 -> Out Bus Element3/1
  Convert_tau_out/1 -> Out Bus Element4/1

== system pmsm_control/Controller/PMSM_FOC/Clarke Transform ==
  Iabc : Inport
  2ib : Gain  Gain=single(2)
  ia : Selector  InputPortWidth=3  IndexOptions=Index vector (dialog)  Indices=1  OutputSizes=1
  ia_plus_2ib : Sum
  ib : Selector  InputPortWidth=3  IndexOptions=Index vector (dialog)  Indices=2  OutputSizes=1
  one_over_sqrt3 : Gain  Gain=single(1/sqrt(3))
  Ialpha : Outport
  Ibeta : Outport  Port=2
  wires:
  one_over_sqrt3/1 -> Ibeta/1
  ia_plus_2ib/1 -> one_over_sqrt3/1
  2ib/1 -> ia_plus_2ib/2
  ib/1 -> 2ib/1
  ia/1 -> ia_plus_2ib/1, Ialpha/1
  Iabc/1 -> ib/1, ia/1

== system pmsm_control/Controller/PMSM_FOC/Electrical Angle ==
  theta_mech : Inport
  pole_pairs : Gain  Gain=single(pp)
  theta_e : Outport
  wires:
  pole_pairs/1 -> theta_e/1
  theta_mech/1 -> pole_pairs/1

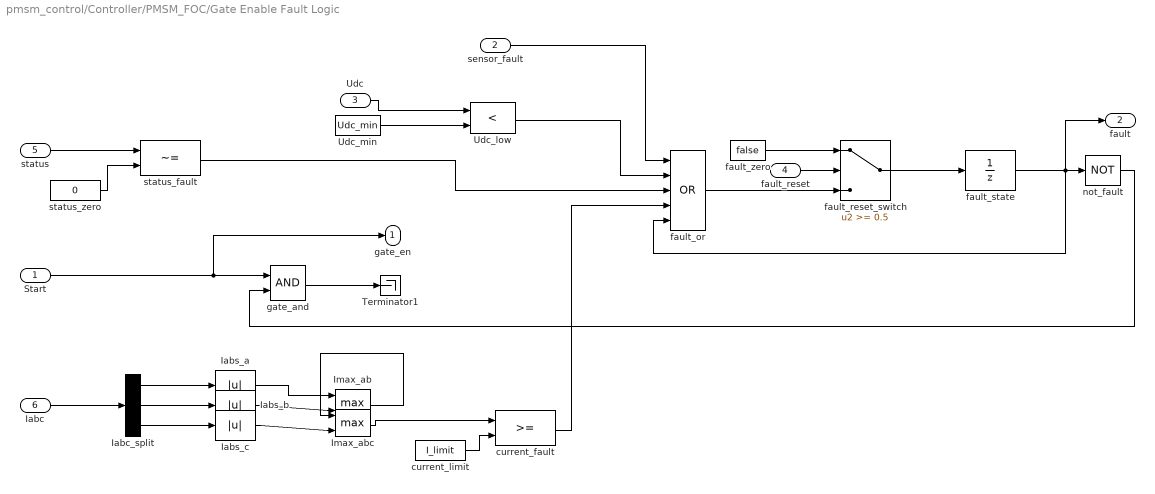
== system pmsm_control/Controller/PMSM_FOC/Gate Enable Fault Logic ==
  Start : Inport
  sensor_fault : Inport  Port=2
  Udc : Inport  Port=3
  fault_reset : Inport  Port=4
  status : Inport  Port=5
  Iabc : Inport  Port=6
  Iabc_split : Demux  Outputs=3
  Iabs_a : Abs
  Iabs_b : Abs
  Iabs_c : Abs
  Imax_ab : MinMax  Function=max  Inputs=2
  Imax_abc : MinMax  Function=max  Inputs=2
  Terminator1 : Terminator
  Udc_low : RelationalOperator  Operator=<  OutDataTypeStr=boolean  RndMeth=Simplest
  Udc_min : Constant  Value=Udc_min  OutDataTypeStr=single  SampleTime=-1
  current_fault : RelationalOperator  OutDataTypeStr=boolean  RndMeth=Simplest
  current_limit : Constant  Value=I_limit  SampleTime=-1
  fault_or : Logic  Operator=OR  Inputs=5  AllPortsSameDT=off  OutDataTypeStr=boolean
  fault_reset_switch : Switch  Threshold=0.5
  fault_state : UnitDelay  InitialCondition=false  SampleTime=-1
  fault_zero : Constant  Value=false  SampleTime=-1
  gate_and : Logic  AllPortsSameDT=off  OutDataTypeStr=boolean
  not_fault : Logic  Operator=NOT  AllPortsSameDT=off  OutDataTypeStr=boolean
  status_fault : RelationalOperator  Operator=~=  OutDataTypeStr=boolean  RndMeth=Simplest
  status_zero : Constant  Value=0  SampleTime=-1
  gate_en : Outport
  fault : Outport  Port=2
  wires:
  status_zero/1 -> status_fault/2
  status/1 -> status_fault/1
  current_limit/1 -> current_fault/2
  Imax_abc/1 -> current_fault/1
  Iabs_c/1 -> Imax_abc/2
  Imax_ab/1 -> Imax_abc/1
  Iabs_b/1 -> Imax_ab/2
  Iabs_a/1 -> Imax_ab/1
  Iabc_split/3 -> Iabs_c/1
  Iabc_split/2 -> Iabs_b/1
  Iabc_split/1 -> Iabs_a/1
  Iabc/1 -> Iabc_split/1
  not_fault/1 -> gate_and/2
  fault_reset_switch/1 -> fault_state/1
  fault_reset/1 -> fault_reset_switch/2
  fault_zero/1 -> fault_reset_switch/1
  fault_or/1 -> fault_reset_switch/3
  current_fault/1 -> fault_or/4
  Udc_low/1 -> fault_or/2
  sensor_fault/1 -> fault_or/1
  Start/1 -> gate_and/1, gate_en/1
  status_fault/1 -> fault_or/3
  gate_and/1 -> Terminator1/1
  Udc_min/1 -> Udc_low/2
  Udc/1 -> Udc_low/1
  fault_state/1 -> fault/1, not_fault/1, fault_or/5

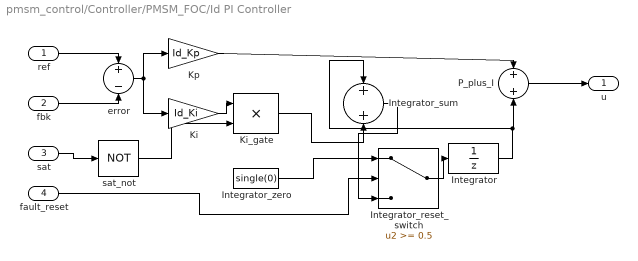
== system pmsm_control/Controller/PMSM_FOC/Id PI Controller ==
  ref : Inport
  fbk : Inport  Port=2
  sat : Inport  Port=3
  fault_reset : Inport  Port=4
  Integrator : UnitDelay  InitialCondition=single(0)  SampleTime=-1
  Integrator_reset_switch : Switch  Threshold=0.5
  Integrator_sum : Sum
  Integrator_zero : Constant  Value=single(0)
  Ki : Gain  Gain=Id_Ki
  Ki_gate : Product  Inputs=**
  Kp : Gain  Gain=Id_Kp
  P_plus_I : Sum
  error : Sum  Inputs=+-
  sat_not : Logic  Operator=NOT  AllPortsSameDT=off  OutDataTypeStr=boolean
  u : Outport
  wires:
  Integrator_reset_switch/1 -> Integrator/1
  Integrator_sum/1 -> Integrator_reset_switch/3
  Integrator_zero/1 -> Integrator_reset_switch/1
  Integrator/1 -> P_plus_I/2, Integrator_sum/1
  sat_not/1 -> Ki_gate/2
  Ki/1 -> Ki_gate/1
  sat/1 -> sat_not/1
  fault_reset/1 -> Integrator_reset_switch/2
  Ki_gate/1 -> Integrator_sum/2
  P_plus_I/1 -> u/1
  Kp/1 -> P_plus_I/1
  error/1 -> Ki/1, Kp/1
  fbk/1 -> error/2
  ref/1 -> error/1

== system pmsm_control/Controller/PMSM_FOC/Inverse Park ==
  Vd : Inport
  Vq : Inport  Port=2
  theta_e : Inport  Port=3
  Valpha_sum : Sum  Inputs=+-
  Vbeta_sum : Sum
  Vd_cos : Product  Inputs=**
  Vd_sin : Product  Inputs=**
  Vq_cos : Product  Inputs=**
  Vq_sin : Product  Inputs=**
  cos : Trigonometry  Operator=cos
  sin : Trigonometry
  Valpha : Outport
  Vbeta : Outport  Port=2
  wires:
  Vbeta_sum/1 -> Vbeta/1
  Valpha_sum/1 -> Valpha/1
  Vq_cos/1 -> Vbeta_sum/2
  Vd_sin/1 -> Vbeta_sum/1
  Vq_sin/1 -> Valpha_sum/2
  Vd_cos/1 -> Valpha_sum/1
  sin/1 -> Vd_sin/2, Vq_sin/2
  Vq/1 -> Vq_cos/1, Vq_sin/1
  cos/1 -> Vq_cos/2, Vd_cos/2
  Vd/1 -> Vd_sin/1, Vd_cos/1
  theta_e/1 -> sin/1, cos/1

== system pmsm_control/Controller/PMSM_FOC/Iq PI Controller ==
  ref : Inport
  fbk : Inport  Port=2
  sat : Inport  Port=3
  fault_reset : Inport  Port=4
  Integrator : UnitDelay  InitialCondition=single(0)  SampleTime=-1
  Integrator_reset_switch : Switch  Threshold=0.5
  Integrator_sum : Sum
  Integrator_zero : Constant  Value=single(0)
  Ki : Gain  Gain=Iq_Ki
  Ki_gate : Product  Inputs=**
  Kp : Gain  Gain=Iq_Kp
  P_plus_I : Sum
  error : Sum  Inputs=+-
  sat_not : Logic  Operator=NOT  AllPortsSameDT=off  OutDataTypeStr=boolean
  u : Outport
  wires:
  Integrator_sum/1 -> Integrator_reset_switch/3
  fault_reset/1 -> Integrator_reset_switch/2
  Integrator_zero/1 -> Integrator_reset_switch/1
  Ki_gate/1 -> Integrator_sum/2
  Integrator/1 -> Integrator_sum/1, P_plus_I/2
  sat_not/1 -> Ki_gate/2
  Ki/1 -> Ki_gate/1
  sat/1 -> sat_not/1
  Integrator_reset_switch/1 -> Integrator/1
  P_plus_I/1 -> u/1
  Kp/1 -> P_plus_I/1
  error/1 -> Kp/1, Ki/1
  fbk/1 -> error/2
  ref/1 -> error/1

== system pmsm_control/Controller/PMSM_FOC/Park Transform ==
  Ialpha : Inport
  Ibeta : Inport  Port=2
  theta_e : Inport  Port=3
  Ialpha_cos : Product  Inputs=**
  Ialpha_sin : Product  Inputs=**
  Ibeta_cos : Product  Inputs=**
  Ibeta_sin : Product  Inputs=**
  Id_sum : Sum
  Iq_sum : Sum  Inputs=+-
  WriteIdMon : DataStoreWrite  DataStoreName=Id_mon
  WriteIqMon : DataStoreWrite  DataStoreName=Iq_mon
  cos : Trigonometry  Operator=cos
  sin : Trigonometry
  Id : Outport
  Iq : Outport  Port=2
  wires:
  Iq_sum/1 -> WriteIqMon/1, Iq/1
  Id_sum/1 -> WriteIdMon/1, Id/1
  Ialpha_sin/1 -> Iq_sum/2
  Ibeta_cos/1 -> Iq_sum/1
  Ibeta_sin/1 -> Id_sum/2
  Ialpha_cos/1 -> Id_sum/1
  sin/1 -> Ialpha_sin/2, Ibeta_sin/2
  Ibeta/1 -> Ibeta_cos/1, Ibeta_sin/1
  cos/1 -> Ibeta_cos/2, Ialpha_cos/2
  Ialpha/1 -> Ialpha_sin/1, Ialpha_cos/1
  theta_e/1 -> sin/1, cos/1

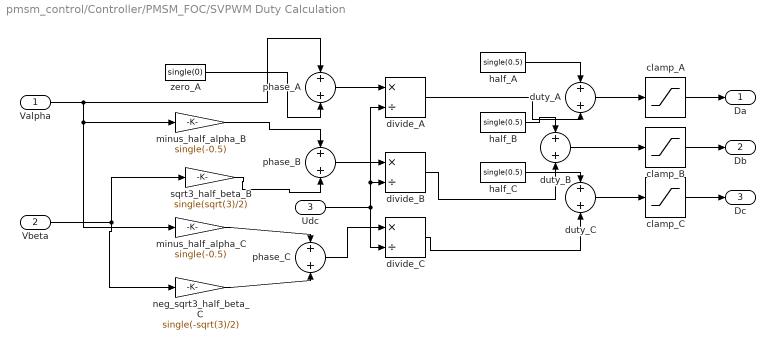
== system pmsm_control/Controller/PMSM_FOC/SVPWM Duty Calculation ==
  Valpha : Inport
  Vbeta : Inport  Port=2
  Udc : Inport  Port=3
  clamp_A : Saturate  UpperLimit=single(1)  LowerLimit=single(0)
  clamp_B : Saturate  UpperLimit=single(1)  LowerLimit=single(0)
  clamp_C : Saturate  UpperLimit=single(1)  LowerLimit=single(0)
  divide_A : Product  Inputs=*/
  divide_B : Product  Inputs=*/
  divide_C : Product  Inputs=*/
  duty_A : Sum
  duty_B : Sum
  duty_C : Sum
  half_A : Constant  Value=single(0.5)  OutDataTypeStr=single  SampleTime=-1
  half_B : Constant  Value=single(0.5)  OutDataTypeStr=single  SampleTime=-1
  half_C : Constant  Value=single(0.5)  OutDataTypeStr=single  SampleTime=-1
  minus_half_alpha_B : Gain  Gain=single(-0.5)
  minus_half_alpha_C : Gain  Gain=single(-0.5)
  neg_sqrt3_half_beta_C : Gain  Gain=single(-sqrt(3)/2)
  phase_A : Sum
  phase_B : Sum
  phase_C : Sum
  sqrt3_half_beta_B : Gain  Gain=single(sqrt(3)/2)
  zero_A : Constant  Value=single(0)  OutDataTypeStr=single  SampleTime=-1
  Da : Outport
  Db : Outport  Port=2
  Dc : Outport  Port=3
  wires:
  clamp_C/1 -> Dc/1
  duty_C/1 -> clamp_C/1
  divide_C/1 -> duty_C/2
  half_C/1 -> duty_C/1
  phase_C/1 -> divide_C/1
  neg_sqrt3_half_beta_C/1 -> phase_C/2
  minus_half_alpha_C/1 -> phase_C/1
  clamp_B/1 -> Db/1
  duty_B/1 -> clamp_B/1
  divide_B/1 -> duty_B/2
  half_B/1 -> duty_B/1
  phase_B/1 -> divide_B/1
  sqrt3_half_beta_B/1 -> phase_B/2
  minus_half_alpha_B/1 -> phase_B/1
  Vbeta/1 -> neg_sqrt3_half_beta_C/1, sqrt3_half_beta_B/1
  clamp_A/1 -> Da/1
  duty_A/1 -> clamp_A/1
  divide_A/1 -> duty_A/2
  half_A/1 -> duty_A/1
  Udc/1 -> divide_A/2, divide_B/2, divide_C/2
  phase_A/1 -> divide_A/1
  zero_A/1 -> phase_A/2
  Valpha/1 -> minus_half_alpha_C/1, minus_half_alpha_B/1, phase_A/1

== system pmsm_control/Controller/PMSM_FOC/Voltage Limit Anti-Windup ==
  Vd_raw : Inport
  Vq_raw : Inport  Port=2
  Udc : Inport  Port=3
  Limit Vd : simulink/Discontinuities/Saturation Dynamic  OutMin=[]  OutMax=[]  OutDataTypeStr=Inherit: Same as second input  OutDataType=fixdt(1, 16)  OutScaling=2^-10  DoSatur=off
  Limit Vq : simulink/Discontinuities/Saturation Dynamic  OutMin=[]  OutMax=[]  OutDataTypeStr=Inherit: Same as second input  OutDataType=fixdt(1, 16)  OutScaling=2^-10  DoSatur=off
  modulation_limit : Gain  Gain=modulation_limit
  neg_limit : Gain  Gain=single(-1)
  sat_or : Logic  Operator=OR  AllPortsSameDT=off  OutDataTypeStr=boolean
  sat_vd : RelationalOperator  Operator=~=  OutDataTypeStr=boolean  RndMeth=Simplest
  sat_vq : RelationalOperator  Operator=~=  OutDataTypeStr=boolean  RndMeth=Simplest
  Vd : Outport
  Vq : Outport  Port=2
  sat : Outport  Port=3
  wires:
  sat_or/1 -> sat/1
  sat_vq/1 -> sat_or/2
  sat_vd/1 -> sat_or/1
  Vd_raw/1 -> sat_vd/1, Limit Vd/2
  modulation_limit/1 -> Limit Vd/1, Limit Vq/1, neg_limit/1
  neg_limit/1 -> Limit Vd/3, Limit Vq/3
  Limit Vd/1 -> sat_vd/2, Vd/1
  Vq_raw/1 -> sat_vq/1, Limit Vq/2
  Limit Vq/1 -> sat_vq/2, Vq/1
  Udc/1 -> modulation_limit/1

== system pmsm_control/Plant/Plant_PMSM_HIL/Bridge ==
  Udc : Inport
  GH : Inport  Port=2
  GL : Inport  Port=3
  Iabc : Inport  Port=4
  AND : Logic  IconShape=distinctive  AllPortsSameDT=off  OutDataTypeStr=boolean
  Compare To Zero : simulink/Logic and Bit Operations/Compare To Zero  relop=<  OutDataTypeStr=boolean
  Constant1 : Constant  Value=0  OutDataTypeStr=Inherit: Inherit via back propagation  SampleTime=-1
  Constant2 : Constant  Value=0  OutDataTypeStr=Inherit: Inherit via back propagation  SampleTime=-1
  NOT : Logic  Operator=NOT  IconShape=distinctive  AllPortsSameDT=off  OutDataTypeStr=boolean
  OR : Logic  Operator=OR  IconShape=distinctive  AllPortsSameDT=off  OutDataTypeStr=boolean
  Sum of Elements : Sum  Inputs=+  OutMax=[ImaxFX]  OutDataTypeStr=fixdt(1,vbits)
  Switch : Switch  Criteria=u2 > Threshold
  Switch1 : Switch  Criteria=u2 > Threshold
  Idc : Outport
  Vabc : Outport  Port=2
  wires:
  Udc/1 -> Switch/1
  Switch/1 -> Vabc/1
  GH/1 -> OR/1
  Switch1/1 -> Sum of Elements/1
  NOT/1 -> AND/1
  Sum of Elements/1 -> Idc/1
  AND/1 -> OR/2
  Iabc/1 -> Compare To Zero/1, Switch1/1
  GL/1 -> NOT/1
  Constant1/1 -> Switch/3
  Compare To Zero/1 -> AND/2
  OR/1 -> Switch1/2, Switch/2
  Constant2/1 -> Switch1/3

== system pmsm_control/Plant/Plant_PMSM_HIL/Clarke ==
  abc : Inport
  1/sqrt(3)1 : Gain  Gain=1/sqrt(3)  ParamDataTypeStr=fixdt(1,cbits)  OutDataTypeStr=Inherit: Same as input
  1/sqrt(3)2 : Gain  Gain=2/3  ParamDataTypeStr=fixdt(1,cbits)  OutDataTypeStr=Inherit: Same as input
  1/sqrt(3)3 : Gain  Gain=1/3  ParamDataTypeStr=fixdt(1,cbits)  OutDataTypeStr=Inherit: Same as input
  Demux : Demux  Outputs=3
  Real-Imag to Complex : RealImagToComplex
  Sum : Sum  Inputs=|+-  OutDataTypeStr=Inherit: Same as accumulator
  Sum1 : Sum  Inputs=|++  OutDataTypeStr=Inherit: Same as accumulator
  Sum2 : Sum  Inputs=|+-  OutDataTypeStr=Inherit: Same as accumulator
  xy : Outport
  wires:
  1/sqrt(3)3/1 -> Sum2/2
  Real-Imag to Complex/1 -> xy/1
  abc/1 -> Demux/1
  Sum2/1 -> Real-Imag to Complex/1
  Demux/1 -> 1/sqrt(3)2/1
  Sum1/1 -> 1/sqrt(3)3/1
  1/sqrt(3)2/1 -> Sum2/1
  Sum/1 -> 1/sqrt(3)1/1
  Demux/2 -> Sum1/1, Sum/1
  1/sqrt(3)1/1 -> Real-Imag to Complex/2
  Demux/3 -> Sum1/2, Sum/2

== system pmsm_control/Plant/Plant_PMSM_HIL/TorqueFromIdq ==
  Idq : Inport
  IdIq : Product
  IdqSplit : ComplexToRealImag
  PMTorqueGain : Gain  Gain=single(1.5*pp*Psi_PM)  OutDataTypeStr=Inherit: Same as input
  RelTorqueGain : Gain  Gain=single(1.5*pp*(Ld-Lq))  OutDataTypeStr=Inherit: Same as input
  TorqueSum : Sum
  tau : Outport
  wires:
  Idq/1 -> IdqSplit/1
  IdqSplit/2 -> PMTorqueGain/1, IdIq/2
  IdqSplit/1 -> IdIq/1
  IdIq/1 -> RelTorqueGain/1
  PMTorqueGain/1 -> TorqueSum/1
  RelTorqueGain/1 -> TorqueSum/2
  TorqueSum/1 -> tau/1

== system pmsm_control/Plant/Plant_PMSM_HIL/invClarke ==
  xy : Inport
  1/sqrt(3)2 : Gain  Gain=sqrt(3)/2  ParamDataTypeStr=fixdt(1,cbits)  OutDataTypeStr=Inherit: Same as input
  Complex to Real-Imag : ComplexToRealImag
  Mux : Mux  Inputs=3
  Shift Arithmetic : ArithShift  BitShiftNumber=1  BitShiftDirection=Right
  Sum : Sum  Inputs=|-+  OutDataTypeStr=Inherit: Same as accumulator
  Sum1 : Sum  Inputs=|--  OutDataTypeStr=Inherit: Same as accumulator
  abc : Outport
  wires:
  Complex to Real-Imag/1 -> Shift Arithmetic/1, Mux/1
  Shift Arithmetic/1 -> Sum/1, Sum1/1
  Sum/1 -> Mux/2
  Sum1/1 -> Mux/3
  1/sqrt(3)2/1 -> Sum1/2, Sum/2
  Complex to Real-Imag/2 -> 1/sqrt(3)2/1
  Mux/1 -> abc/1
  xy/1 -> Complex to Real-Imag/1

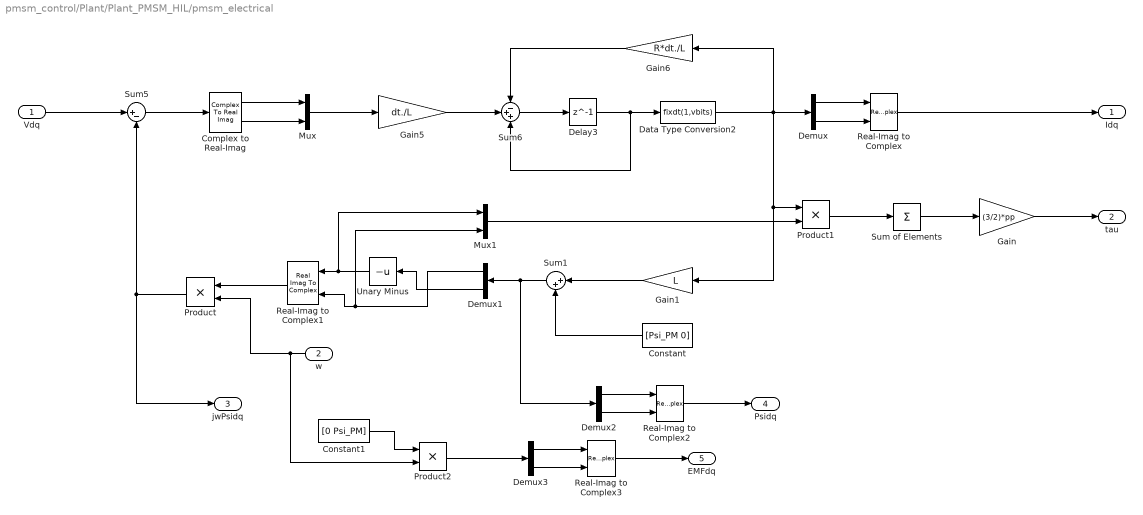
== system pmsm_control/Plant/Plant_PMSM_HIL/pmsm_electrical ==
  Vdq : Inport
  w : Inport  Port=2
  Complex to Real-Imag : ComplexToRealImag
  Constant : Constant  Value=[Psi_PM 0]  OutDataTypeStr=fixdt(1,vbits)  SampleTime=-1
  Constant1 : Constant  Value=[0 Psi_PM]  OutDataTypeStr=fixdt(1,vbits)  SampleTime=-1
  Data Type Conversion2 : DataTypeConversion  OutMax=[ImaxFX]  OutDataTypeStr=fixdt(1,vbits)
  Delay3 : Delay  DelayLength=1  InitialCondition=0
  Demux{,1..3} (4 alike) : Demux  Outputs=2
  Gain : Gain  Gain=(3/2)*pp  ParamDataTypeStr=fixdt(1,cbits)  OutMax=[(3/2)*pp*PsimaxFX*ImaxFX]  OutDataTypeStr=fixdt(1,vbits)
  Gain1 : Gain  Gain=L  ParamDataTypeStr=fixdt(1,cbits)  OutMax=[max(L*ImaxFX)]  OutDataTypeStr=fixdt(1,vbits)
  Gain5 : Gain  Gain=dt./L  ParamDataTypeStr=fixdt(1,cbits)  OutMax=[max(dt./L*UmaxFX)]  OutDataTypeStr=fixdt(1,vbits)
  Gain6 : Gain  Gain=R*dt./L  ParamDataTypeStr=fixdt(1,cbits)  OutMax=[max(R*dt./L)*ImaxFX]  OutDataTypeStr=fixdt(1,vbits)
  Mux : Mux  Inputs=2
  Mux1 : Mux  Inputs=2
  Product : Product  OutMax=[UmaxFX]  OutDataTypeStr=fixdt(1,vbits)
  Product1 : Product  OutMax=[ImaxFX*PsimaxFX]  OutDataTypeStr=fixdt(1,vbits)
  Product2 : Product  OutMax=[UmaxFX]  OutDataTypeStr=fixdt(1,vbits)
  Real-Imag to Complex{,1..3} (4 alike) : RealImagToComplex
  Sum of Elements : Sum  Inputs=+  OutDataTypeStr=Inherit: Same as accumulator
  Sum1 : Sum  Inputs=|++  OutDataTypeStr=Inherit: Same as accumulator
  Sum5 : Sum  Inputs=|+-  OutDataTypeStr=Inherit: Same as accumulator
  Sum6 : Sum  Inputs=-++  OutDataTypeStr=fixdt(1,44,33)
  Unary Minus : UnaryMinus
  Idq : Outport
  tau : Outport  Port=2
  jwPsidq : Outport  Port=3
  Psidq : Outport  Port=4
  EMFdq : Outport  Port=5
  wires:
  Real-Imag to Complex/1 -> Idq/1
  Real-Imag to Complex1/1 -> Product/1
  Sum of Elements/1 -> Gain/1
  Mux1/1 -> Product1/2
  Sum5/1 -> Complex to Real-Imag/1
  Complex to Real-Imag/2 -> Mux/2
  Vdq/1 -> Sum5/1
  w/1 -> Product2/2, Product/2
  Complex to Real-Imag/1 -> Mux/1
  Unary Minus/1 -> Real-Imag to Complex1/1, Mux1/1
  Gain6/1 -> Sum6/1
  Product/1 -> jwPsidq/1, Sum5/2
  Gain1/1 -> Sum1/1
  Product1/1 -> Sum of Elements/1
  Demux1/1 -> Real-Imag to Complex1/2, Mux1/2
  Constant/1 -> Sum1/2
  Demux/2 -> Real-Imag to Complex/2
  Delay3/1 -> Sum6/3, Data Type Conversion2/1
  Demux/1 -> Real-Imag to Complex/1
  Demux1/2 -> Unary Minus/1
  Data Type Conversion2/1 -> Gain6/1, Demux/1, Gain1/1, Product1/1
  Mux/1 -> Gain5/1
  Gain/1 -> tau/1
  Sum6/1 -> Delay3/1
  Gain5/1 -> Sum6/2
  Sum1/1 -> Demux2/1, Demux1/1
  Demux2/1 -> Real-Imag to Complex2/1
  Demux2/2 -> Real-Imag to Complex2/2
  Real-Imag to Complex2/1 -> Psidq/1
  Demux3/2 -> Real-Imag to Complex3/2
  Demux3/1 -> Real-Imag to Complex3/1
  Product2/1 -> Demux3/1
  Real-Imag to Complex3/1 -> EMFdq/1
  Constant1/1 -> Product2/1

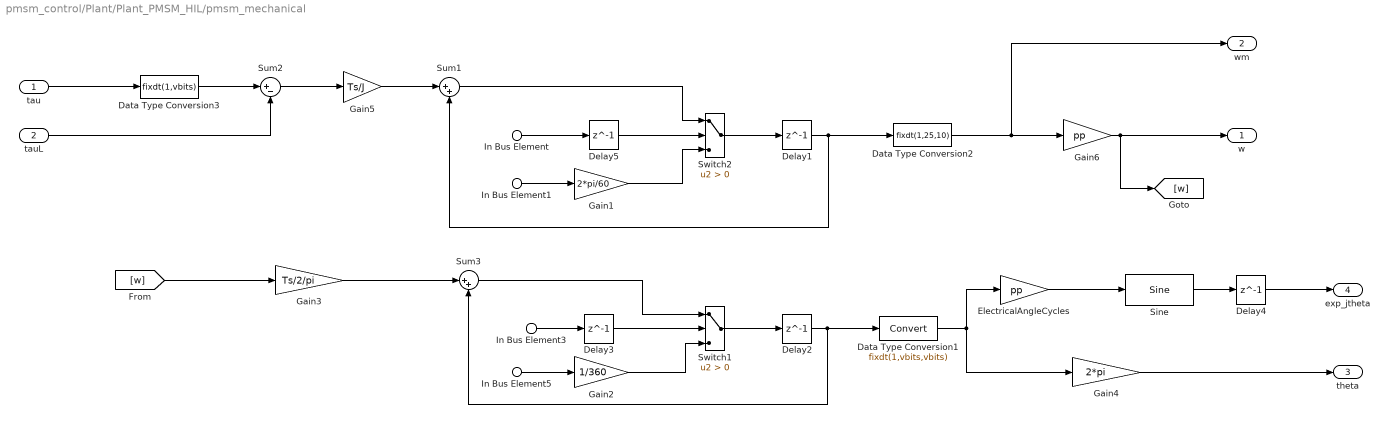
== system pmsm_control/Plant/Plant_PMSM_HIL/pmsm_mechanical ==
  tau : Inport
  tauL : Inport  Port=2
  In Bus Element : Inport  Port=3  PortName=p  Element=speed_en
  In Bus Element1 : Inport  Port=3  PortName=p  Element=speed0
  In Bus Element3 : Inport  Port=3  PortName=p  Element=theta_en
  In Bus Element5 : Inport  Port=3  PortName=p  Element=theta0
  Data Type Conversion1 : DataTypeConversion  OutDataTypeStr=fixdt(1,vbits,vbits)
  Data Type Conversion2 : DataTypeConversion  OutMax=[WmaxFX/pp]  OutDataTypeStr=fixdt(1,25,10)
  Data Type Conversion3 : DataTypeConversion  OutMax=[TaumaxFX]  OutDataTypeStr=fixdt(1,vbits)
  Delay{1..5} (5 alike) : Delay  DelayLength=1  InitialCondition=0
  ElectricalAngleCycles : Gain  Gain=pp  OutDataTypeStr=fixdt(1,26,25)
  Gain1 : Gain  Gain=2*pi/60  ParamDataTypeStr=fixdt(1,cbits)  OutMax=[WmaxFX/pp]  OutDataTypeStr=fixdt(1,25,10)
  Gain2 : Gain  Gain=1/360  OutMax=[0.5]  OutDataTypeStr=fixdt(1,26,25)
  Gain3 : Gain  Gain=Ts/2/pi  ParamDataTypeStr=fixdt(1,cbits)  OutMax=[WmaxFX*dt/2/pi]  OutDataTypeStr=fixdt(1,38,38)
  Gain4 : Gain  Gain=2*pi  ParamDataTypeStr=fixdt(1,cbits)  OutMax=[pi]  OutDataTypeStr=fixdt(1,25,20)
  Gain5 : Gain  Gain=Ts/J  ParamDataTypeStr=fixdt(1,cbits)  OutMax=[dt/J*TaumaxFX]  OutDataTypeStr=fixdt(1,49,37)
  Gain6 : Gain  Gain=pp  OutMax=[WmaxFX]  OutDataTypeStr=fixdt(1,25,10)
  Sine : simulink/Lookup Tables/Sine  Formula=exp(j*2*pi*u)  NumDataPoints=(2^5)+1  OutputWordLength=16  InternalRulePriority=Speed
      settings: SourceProductName=Simulink
  Sum1 : Sum  Inputs=|++  OutDataTypeStr=fixdt(1,12+37,37)
  Sum2 : Sum  Inputs=|+-  OutDataTypeStr=Inherit: Same as accumulator
  Sum3 : Sum  Inputs=|++  OutDataTypeStr=fixdt(1,38,38)
  Switch1 : Switch  Criteria=u2 > Threshold  OutDataTypeStr=fixdt(1,38,38)
  Switch2 : Switch  Criteria=u2 > Threshold  OutDataTypeStr=fixdt(1,49,37)
  w : Outport
  wm : Outport  Port=2
  theta : Outport  Port=3
  exp_jtheta : Outport  Port=4
  wires:
  Gain4/1 -> theta/1
  Data Type Conversion3/1 -> Sum2/1
  Data Type Conversion1/1 -> Gain4/1, ElectricalAngleCycles/1
  Data Type Conversion2/1 -> Gain6/1, wm/1
  [w] -> Gain3/1
  In Bus Element5/1 -> Gain2/1
  In Bus Element3/1 -> Delay3/1
  Switch1/1 -> Delay2/1
  Gain2/1 -> Switch1/3
  Delay3/1 -> Switch1/2
  Sum3/1 -> Switch1/1
  Delay2/1 -> Sum3/2, Data Type Conversion1/1
  Gain3/1 -> Sum3/1
  Gain1/1 -> Switch2/3
  In Bus Element/1 -> Delay5/1
  In Bus Element1/1 -> Gain1/1
  Switch2/1 -> Delay1/1
  Delay5/1 -> Switch2/2
  Gain5/1 -> Sum1/1
  Sum1/1 -> Switch2/1
  tau/1 -> Data Type Conversion3/1
  Gain6/1 -> [w], w/1
  tauL/1 -> Sum2/2
  Delay1/1 -> Sum1/2, Data Type Conversion2/1
  Sum2/1 -> Gain5/1
  Sine/1 -> Delay4/1
  Delay4/1 -> exp_jtheta/1
  ElectricalAngleCycles/1 -> Sine/1

== stateflow chart pmsm_control/Scheduler/AsynchronousScheduler ==
  settings: executeAtInitialization=1
  state AsynchronousScheduler
    AsynchronousScheduler -> (junction 6) : pwm_it { send(adc_it); }
  events: pwm_it input RISING_EDGE_EVENT; adc_it output FUNCTION_CALL_EVENT
